simulink model "Schema_Y_Q2"  (R2025b)
settings: Solver=VariableStepAuto  StartTime=0.0  StopTime=10.0  RelTol=1e-3
values from neighbouring files (symbols this model uses):
  Kdy = 15000    [script_devoir2.m]
  Kiy = 125000    [script_devoir2.m]
  Kpy = 75000    [script_devoir2.m]
  m = 1000    [script_devoir2.m]
settings Model: Creator=Louis  LastModifiedBy=Louis

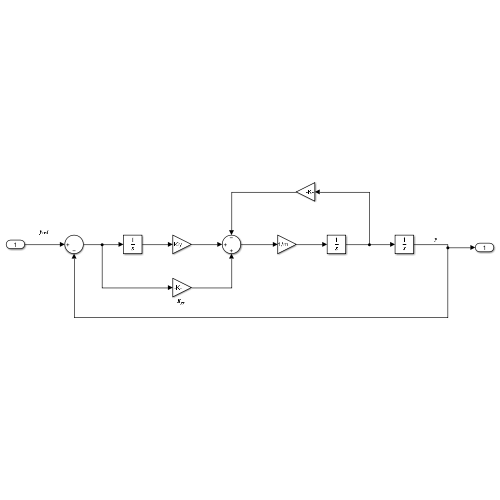
[thumbnail: Simulink's stored preview of the top-level diagram]
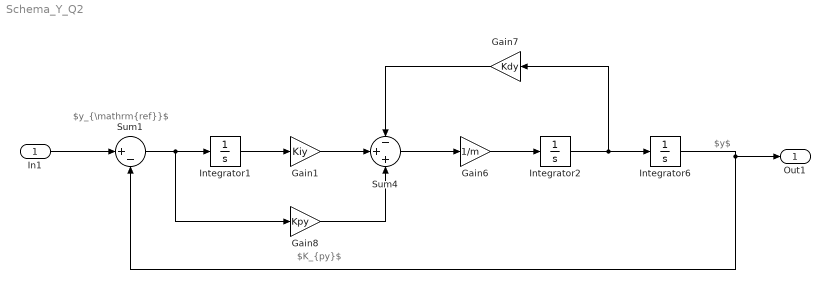
== system Schema_Y_Q2 ==
  note: $y_{\mathrm{ref}}$
  note: $y$
  note: $K_{py}$
  In1 : Inport
  Gain1 : Gain  Gain=Kiy
  Gain6 : Gain  Gain=1/m
  Gain7 : Gain  Gain=Kdy
  Gain8 : Gain  Gain=Kpy
  Integrator1 : Integrator
  Integrator2 : Integrator
  Integrator6 : Integrator
  Sum1 : Sum  Inputs=|+-
  Sum4 : Sum  Inputs=-++
  Out1 : Outport
  wires:
  Gain8/1 -> Sum4/3
  Gain7/1 -> Sum4/1
  Sum4/1 -> Gain6/1
  In1/1 -> Sum1/1
  Integrator2/1 -> Gain7/1, Integrator6/1
  Integrator6/1 -> Out1/1, Sum1/2
  Gain6/1 -> Integrator2/1
  Sum1/1 -> Gain8/1, Integrator1/1
  Integrator1/1 -> Gain1/1
  Gain1/1 -> Sum4/2
